simulink library "INT_RmtAPP_PlausBrk"  (R2016b)
settings: Solver=VariableStepAuto  StartTime=0.0  StopTime=10.0  RelTol=1e-3
settings Model: Creator=bianxuyin  LastModifiedBy=bianxuyin

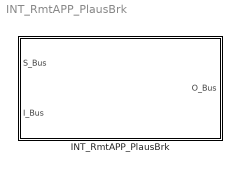
== system INT_RmtAPP_PlausBrk ==
  INT_RmtAPP_PlausBrk : Subsystem

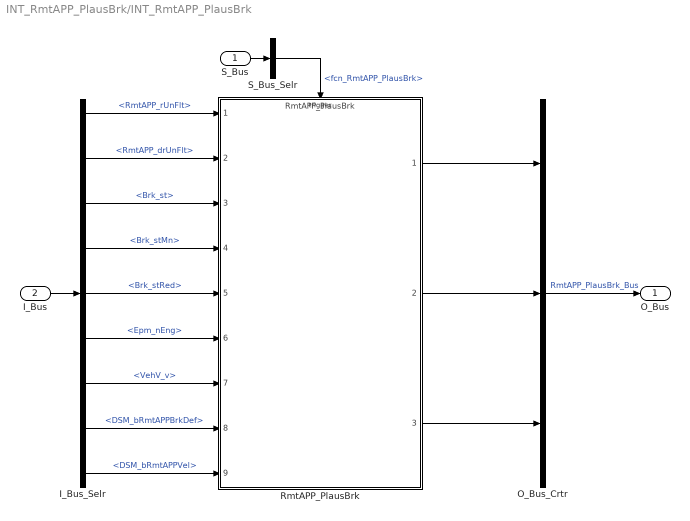
== system INT_RmtAPP_PlausBrk/INT_RmtAPP_PlausBrk ==
  S_Bus : Inport
  I_Bus : Inport  Port=2
  I_Bus_Selr : BusSelector  OutputSignals=RmtAPP_rUnFlt,RmtAPP_drUnFlt,Brk_st,Brk_stMn,Brk_stRed,Epm_nEng,VehV_v,DSM_bRmtAPPBrkDef,DSM_bRmtAPPVel
  O_Bus_Crtr : BusCreator  Inputs=3
  RmtAPP_PlausBrk : ModelReference  ModelNameDialog=RmtAPP_PlausBrk  SimulationMode=Normal  ModelReferenceVersion=1.8  TriggerPortName=function  TriggerPortTriggerType=function-call  TriggerPortStatesWhenEnabling=held
  S_Bus_Selr : BusSelector  OutputSignals=fcn_RmtAPP_PlausBrk
  O_Bus : Outport
  wires:
  S_Bus_Selr/1 -> RmtAPP_PlausBrk/Trigger  "<fcn_RmtAPP_PlausBrk>"
  S_Bus/1 -> S_Bus_Selr/1
  I_Bus/1 -> I_Bus_Selr/1
  I_Bus_Selr/1 -> RmtAPP_PlausBrk/1  "<RmtAPP_rUnFlt>"
  I_Bus_Selr/2 -> RmtAPP_PlausBrk/2  "<RmtAPP_drUnFlt>"
  I_Bus_Selr/3 -> RmtAPP_PlausBrk/3  "<Brk_st>"
  I_Bus_Selr/4 -> RmtAPP_PlausBrk/4  "<Brk_stMn>"
  I_Bus_Selr/5 -> RmtAPP_PlausBrk/5  "<Brk_stRed>"
  I_Bus_Selr/6 -> RmtAPP_PlausBrk/6  "<Epm_nEng>"
  I_Bus_Selr/7 -> RmtAPP_PlausBrk/7  "<VehV_v>"
  I_Bus_Selr/8 -> RmtAPP_PlausBrk/8  "<DSM_bRmtAPPBrkDef>"
  I_Bus_Selr/9 -> RmtAPP_PlausBrk/9  "<DSM_bRmtAPPVel>"
  O_Bus_Crtr/1 -> O_Bus/1  "RmtAPP_PlausBrk_Bus"
  RmtAPP_PlausBrk/1 -> O_Bus_Crtr/1
  RmtAPP_PlausBrk/2 -> O_Bus_Crtr/2
  RmtAPP_PlausBrk/3 -> O_Bus_Crtr/3
